simulink model "ulohaDva_simulink"  (R2022b)
settings: Solver=VariableStepAuto  StartTime=0.0  StopTime=10  RelTol=1e-3
model workspace (MAT data in the model file):
  a0 = -5
  a1 = -4
  a2 = 1
values from neighbouring files (symbols this model uses):
  a = input("Zadaj koeficienty LDR: [a2 a1 a0] = [1 -4 -5]\n")    [main.m]
libraries: simulink x1
settings Model: Creator=marak  LastModifiedBy=marak

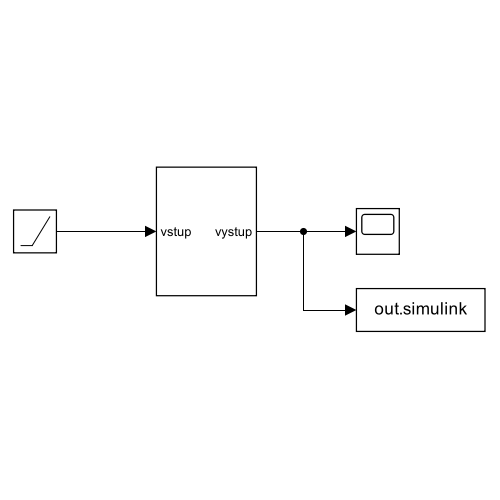
[thumbnail: Simulink's stored preview of the top-level diagram]
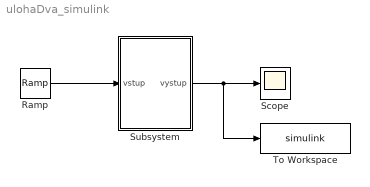
== system ulohaDva_simulink ==
  Ramp : simulink/Sources/Ramp  slope=1  start=t(1)  InitialOutput=t(2)
  Scope : Scope
  Subsystem : Subsystem  mask{a2=a(1), a1=a(2), a0=a(3)}
  To Workspace : ToWorkspace  VariableName=simulink  SaveFormat=Timeseries  SampleTime=-1
  wires:
  Ramp/1 -> Subsystem/1(vstup)
  Subsystem/1(vystup) -> To Workspace/1, Scope/1

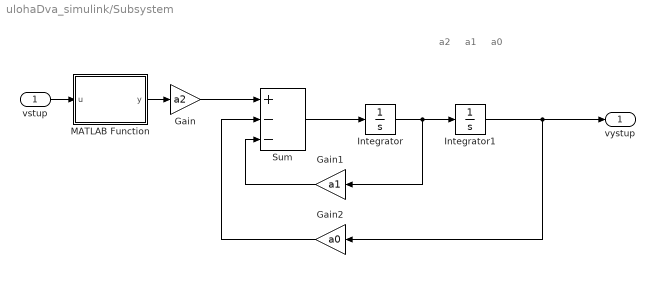
== system ulohaDva_simulink/Subsystem ==
  note: a0
  note: a1
  note: a2
  vstup : Inport
  Gain : Gain  Gain=a2
  Gain1 : Gain  Gain=a1
  Gain2 : Gain  Gain=a0
  Integrator : Integrator
  Integrator1 : Integrator
  MATLAB Function : MATLAB Function  TreatAsAtomicUnit=on
  Sum : Sum  Inputs=+--
  vystup : Outport
  wires:
  Sum/1 -> Integrator/1
  Integrator1/1 -> vystup/1, Gain2/1
  Gain/1 -> Sum/1
  Integrator/1 -> Gain1/1, Integrator1/1
  MATLAB Function/1(y) -> Gain/1
  Gain1/1 -> Sum/3
  Gain2/1 -> Sum/2
  vstup/1 -> MATLAB Function/1(u)

== matlab function ulohaDva_simulink/Subsystem/MATLAB Function ==
  data: u input; y output
function y = fcn(u)
    y = exp(2*u);
